simulink model "sender"  (R2019b)
settings: Solver=VariableStepAuto  StartTime=0.0  StopTime=10e-3  RelTol=1e-3
values from neighbouring files (symbols this model uses):
  f_c = 100e3    (= 100000)    [loopFil.m]
  filter = rcosdesign(alpha,symNum,sym,'sqrt')    [loopFil.m]    (also in rcosfilter.m)
  Gc = 1    [loopFil.m]
  Gg = 1.5    [loopFil.m]
  inc = 2^16*f_nco/Fs    (= 5688.88888889)    [loopFil.m]
  inc2 = 2^16*f_nco2/Fs    (= 8533.33333333)    [loopFil.m]
  inc_src = 2^16*f_src/Fs    (= 1092.26666667)    [loopFil.m]
undefined symbols (not defined in the file or in its folder): ac, ag, bc, bg, fdesignblkfcn, gcbh
libraries: dspsigops x22, dspsrcs4 x8, simulink x4
settings Model: Creator=Administrator  LastModifiedBy=Administrator

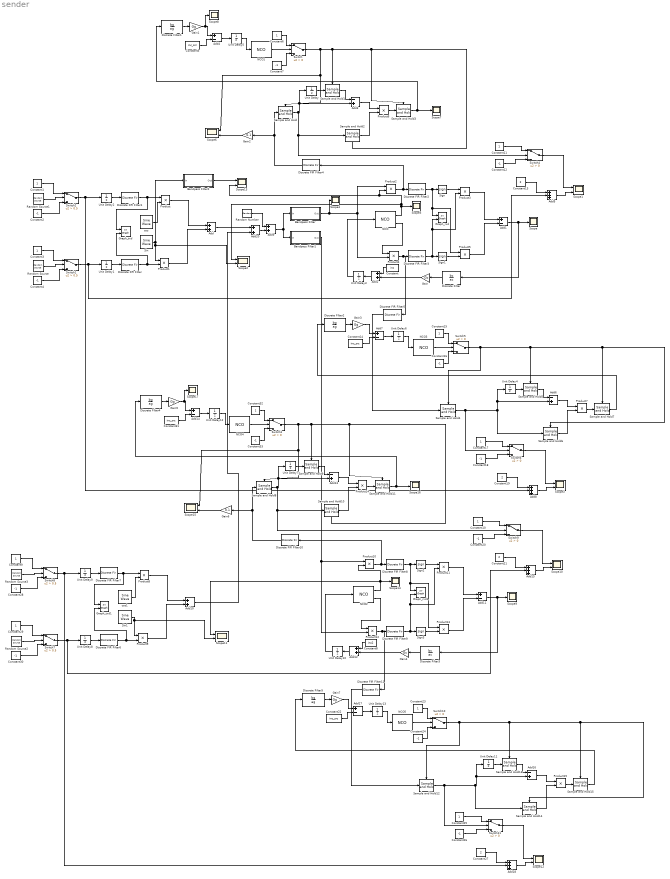
== system sender ==
  Add{,2,10,12} (4 alike) : Sum
  Add1 : Sum  Inputs=+-
  Add11 : Sum  Inputs=+-
  Add{3,6,13,16} (4 alike) : Sum  Inputs=-+
  Add{4,7,14,17} (4 alike) : Sum  Inputs=+-  OutDataTypeStr=int16
  Add{5,8,15,18} (4 alike) : Sum  Inputs=+++  OutDataTypeStr=int16
  Add20 : Sum  OutDataTypeStr=int16
  Add9 : Sum  OutDataTypeStr=int16
  Bandpass Filter : Subsystem  DialogController=fdesignblkfcn  InitFcn=fdesignblkfcn(gcbh, {'InitFcn'});  mask(Bandpass Filter){}
      mask help: Design a bandpass filter
      settings: CopyFcn=fdesignblkfcn(gcbh, {'CopyFcn'});
      mask Help: helpview(mapfilelocation('dsp'), 'dspbandpassfilter');
      mask Display: disp('Bandpass');
  Bandpass Filter1 : Subsystem  DialogController=fdesignblkfcn  InitFcn=fdesignblkfcn(gcbh, {'InitFcn'});  mask(Bandpass Filter){}
      mask help: Design a bandpass filter
      settings: CopyFcn=fdesignblkfcn(gcbh, {'CopyFcn'});
      mask Help: helpview(mapfilelocation('dsp'), 'dspbandpassfilter');
      mask Display: disp('Bandpass');
  Bandpass Filter2 : Subsystem  DialogController=fdesignblkfcn  InitFcn=fdesignblkfcn(gcbh, {'InitFcn'});  mask(Bandpass Filter){}
      mask help: Design a bandpass filter
      settings: CopyFcn=fdesignblkfcn(gcbh, {'CopyFcn'});
      mask Help: helpview(mapfilelocation('dsp'), 'dspbandpassfilter');
      mask Display: disp('Bandpass');
  Constant : Constant  Value=inc  OutDataTypeStr=int16  SampleTime=1/(60*19.2e3)
  Constant{1,3,6,9..11,15,17,23,25,29,32} (12 alike) : Constant  SampleTime=1/(60*19.2e3)
  Constant{2,4,7,12,16,18,20,24,26,28,30,33} (12 alike) : Constant  Value=-1  SampleTime=1/(60*19.2e3)
  Constant{13,19,21,27} (4 alike) : Constant  Value=2  SampleTime=1/(60*19.2e3)
  Constant{5,14,22,31} (4 alike) : Constant  Value=inc_src  OutDataTypeStr=int32  SampleTime=1/(60*19.2e3)
  Constant8 : Constant  Value=inc2  OutDataTypeStr=int16  SampleTime=1/(60*19.2e3)
  Discrete FIR Filter{,1..11} (12 alike) : DiscreteFir  Coefficients=filter
  Discrete Filter : DiscreteFilter  Numerator=bc  Denominator=ac
  Discrete Filter{1..2,4..5} (4 alike) : DiscreteFilter  Numerator=bg  Denominator=ag
  Discrete Filter3 : DiscreteFilter  Numerator=bc  Denominator=ac
  Gain : Gain  Gain=Gc  OutDataTypeStr=int16
  Gain{1,3,5,7} (4 alike) : Gain  Gain=Gg
  Gain2 : Gain  Gain=0.1
  Gain4 : Gain  Gain=Gc  OutDataTypeStr=int16
  Gain6 : Gain  Gain=0.1
  Graph_rxd : simulink/Sinks/XY Graph  xmin=-50  xmax=50  ymin=-50  ymax=50  st=-1
  Graph_rxd1 : simulink/Sinks/XY Graph  xmin=-50  xmax=50  ymin=-50  ymax=50  st=-1
  Graph_txd : simulink/Sinks/XY Graph  xmin=-16  xmax=16  ymin=-16  ymax=16  st=-1
  Graph_txd1 : simulink/Sinks/XY Graph  xmin=-16  xmax=16  ymin=-16  ymax=16  st=-1
  NCO : dspsigops/NCO  AccIncSrc=Input port  AccInc=100  PhaseOffsetSrc=Specify via dialog  PhaseOffset=0  AccumWL=16  HasDither=on  DitherWL=4  PNgeneratorLength=19  HasPhaseQuantizer=on  TableDepth=12  HasOutputPhaseError=off  Formula=Sine and cosine  DataType=single  OutputWL=16  OutputFL=14  CompMethod=Table lookup (no interpolation)  SampleTime=1  SamplesPerFrame=1  OutputFrames=off
      settings: SourceProductName=DSP System Toolbox  SourceProductBaseCode=DS
  NCO{1,3..5} (4 alike) : dspsigops/NCO  AccIncSrc=Input port  AccInc=100  PhaseOffsetSrc=Specify via dialog  PhaseOffset=0  AccumWL=16  HasDither=on  DitherWL=4  PNgeneratorLength=19  HasPhaseQuantizer=on  TableDepth=12  HasOutputPhaseError=off  Formula=Sine  DataType=single  OutputWL=16  OutputFL=14  CompMethod=Table lookup (no interpolation)  SampleTime=1  SamplesPerFrame=1  OutputFrames=off
      settings: SourceProductName=DSP System Toolbox  SourceProductBaseCode=DS
  NCO2 : dspsigops/NCO  AccIncSrc=Input port  AccInc=100  PhaseOffsetSrc=Specify via dialog  PhaseOffset=0  AccumWL=16  HasDither=on  DitherWL=4  PNgeneratorLength=19  HasPhaseQuantizer=on  TableDepth=12  HasOutputPhaseError=off  Formula=Sine and cosine  DataType=single  OutputWL=16  OutputFL=14  CompMethod=Table lookup (no interpolation)  SampleTime=1  SamplesPerFrame=1  OutputFrames=off
      settings: SourceProductName=DSP System Toolbox  SourceProductBaseCode=DS
  Product{,1..15} (16 alike) : Product
  Random Number : RandomNumber  Variance=0  SampleTime=1/(60*19.2e3)
  Random Source{,1..3} (4 alike) : dspsrcs4/Random Source  SrcType=Uniform  NormMethod=Ziggurat  CltLength=12  MinVal=0  MaxVal=1  MeanVal=0  VarVal=1  RepMode=Not repeatable  rawSeed=1  IsInherit=off  SampMode=Discrete  SampTime=1/(19.2e3)  SampFrame=1  DataType=Double  OutComplex=Real  OutputFrames=off
  Sample and Hold{,1,4..5,8..9,12..13} (8 alike) : dspsigops/Sample and Hold  trig=Rising edge  initCond=0  latchinput=off
  Sample and Hold{2,6,10,14} (4 alike) : dspsigops/Sample and Hold  trig=Falling edge  initCond=0  latchinput=off
  Sample and Hold{3,7,11,15} (4 alike) : dspsigops/Sample and Hold  Tag=error  trig=Rising edge  initCond=0  latchinput=off
  Scope{,4..5,7..9,14,16..17} (9 alike) : Scope
  Scope{1..3,6,10..13,15} (9 alike) : Scope  NumInputPorts=2
  Sign{,1..3} (4 alike) : Signum
  Sin : dspsrcs4/Sine Wave  Amplitude=1  Frequency=f_c  Phase=0  SampleMode=Discrete  OutComplex=Real  CompMethod=Trigonometric fcn  TableSize=Speed  SampleTime=1/(60*19.2e3)  SamplesPerFrame=1  ResetState=Restart at time zero  OutputFrames=off  dataType=double  wordLen=16  udDataType=sfix(16)  fracBitsMode=Best precision  numFracBits=15  OutDataTypeStr=double  LastOutDataTypeStr=double
  Sin1 : dspsrcs4/Sine Wave  Amplitude=1  Frequency=150e3  Phase=0  SampleMode=Discrete  OutComplex=Real  CompMethod=Trigonometric fcn  TableSize=Speed  SampleTime=1/(60*19.2e3)  SamplesPerFrame=1  ResetState=Restart at time zero  OutputFrames=off  dataType=double  wordLen=16  udDataType=sfix(16)  fracBitsMode=Best precision  numFracBits=15  OutDataTypeStr=double  LastOutDataTypeStr=double
  Switch{,3..6,9..11} (8 alike) : Switch  Criteria=u2 > Threshold
  Switch{1..2,7..8} (4 alike) : Switch  Criteria=u2 > Threshold  Threshold=0.5
  Unit Delay{,1..13} (14 alike) : UnitDelay  SampleTime=-1  HasFrameUpgradeWarning=on
  cos : dspsrcs4/Sine Wave  Amplitude=1  Frequency=f_c  Phase=pi/2  SampleMode=Discrete  OutComplex=Real  CompMethod=Trigonometric fcn  TableSize=Speed  SampleTime=1/(60*19.2e3)  SamplesPerFrame=1  ResetState=Restart at time zero  OutputFrames=off  dataType=double  wordLen=16  udDataType=sfix(16)  fracBitsMode=Best precision  numFracBits=15  OutDataTypeStr=double  LastOutDataTypeStr=double
  cos1 : dspsrcs4/Sine Wave  Amplitude=1  Frequency=150e3  Phase=pi/2  SampleMode=Discrete  OutComplex=Real  CompMethod=Trigonometric fcn  TableSize=Speed  SampleTime=1/(60*19.2e3)  SamplesPerFrame=1  ResetState=Restart at time zero  OutputFrames=off  dataType=double  wordLen=16  udDataType=sfix(16)  fracBitsMode=Best precision  numFracBits=15  OutDataTypeStr=double  LastOutDataTypeStr=double
  wires:
  Unit Delay1/1 -> Discrete FIR Filter/1
  Discrete FIR Filter/1 -> Graph_txd/2, Product1/2
  Sin/1 -> Bandpass Filter2/1(In), Scope2/2, Product1/1
  cos/1 -> Product/2
  Product/1 -> Add/1
  Product1/1 -> Add/2
  Product3/1 -> Add1/1
  Sign1/1 -> Product5/2
  Product5/1 -> Add1/2
  Discrete FIR Filter2/1 -> Graph_rxd/1, Product5/1, Sign/1
  Discrete FIR Filter3/1 -> Graph_rxd/2, Product3/2, Sign1/1
  Sign/1 -> Product3/1
  Add1/1 -> Discrete Filter/1, Scope/1
  Product2/1 -> Discrete FIR Filter4/1, Discrete FIR Filter2/1
  Product4/1 -> Discrete FIR Filter5/1, Discrete FIR Filter3/1
  NCO/1 -> Scope13/2, Product2/2, Scope2/1, Scope5/1
  NCO/2 -> Product4/1
  Constant/1 -> Add2/1
  Add2/1 -> Unit Delay3/1
  Unit Delay3/1 -> NCO/1
  Sample and Hold/1 -> Sample and Hold2/1, Switch4/2, Unit Delay/1, Add3/2
  Gain1/1 -> Scope8/1, Add4/1
  Switch/1 -> Sample and Hold1/Trigger, Sample and Hold2/Trigger, Sample and Hold3/Trigger, Sample and Hold/Trigger, Scope6/1
  Constant6/1 -> Switch/1
  Sample and Hold1/1 -> Add3/1
  Product6/1 -> Sample and Hold3/1
  Unit Delay5/1 -> NCO1/1
  NCO1/1 -> Switch/2
  Constant5/1 -> Add4/2
  Constant7/1 -> Switch/3
  Unit Delay/1 -> Sample and Hold1/1
  Sample and Hold2/1 -> Product6/2
  Add4/1 -> Unit Delay5/1
  Add3/1 -> Product6/1
  Discrete Filter/1 -> Gain/1
  Gain/1 -> Add2/2
  Discrete Filter1/1 -> Gain1/1
  Sample and Hold3/1 -> Scope7/1, Discrete Filter1/1
  Discrete FIR Filter4/1 -> Sample and Hold/1, Gain2/1
  Constant1/1 -> Switch2/1
  Constant2/1 -> Switch2/3
  Random Source1/1 -> Switch2/2
  Constant3/1 -> Switch1/1
  Constant4/1 -> Switch1/3
  Random Source/1 -> Switch1/2
  Gain2/1 -> Scope6/2
  Switch2/1 -> Add8/2, Unit Delay2/1
  Switch1/1 -> Add5/2, Unit Delay1/1
  Constant11/1 -> Switch4/1
  Constant12/1 -> Switch4/3
  Switch4/1 -> Scope1/1
  Constant13/1 -> Add5/1
  Add5/1 -> Scope1/2
  Constant14/1 -> Add7/2
  Sample and Hold7/1 -> Discrete Filter2/1
  Discrete Filter2/1 -> Gain3/1
  Add7/1 -> Unit Delay6/1
  Discrete FIR Filter5/1 -> Sample and Hold4/1
  Unit Delay4/1 -> Sample and Hold5/1
  Sample and Hold6/1 -> Product7/2
  Product7/1 -> Sample and Hold7/1
  Add6/1 -> Product7/1
  Gain3/1 -> Add7/1
  Constant16/1 -> Switch5/3
  Unit Delay6/1 -> NCO3/1
  Switch5/1 -> Sample and Hold5/Trigger, Sample and Hold6/Trigger, Sample and Hold7/Trigger, Sample and Hold4/Trigger
  NCO3/1 -> Switch5/2
  Sample and Hold4/1 -> Switch6/2, Sample and Hold6/1, Unit Delay4/1, Add6/2
  Sample and Hold5/1 -> Add6/1
  Constant15/1 -> Switch5/1
  Constant18/1 -> Switch6/3
  Switch6/1 -> Scope3/1
  Constant17/1 -> Switch6/1
  Add8/1 -> Scope3/2
  Constant19/1 -> Add8/1
  Random Number/1 -> Add9/1
  Constant24/1 -> Switch10/3
  Constant23/1 -> Switch10/1
  Switch9/1 -> Scope10/1
  Constant10/1 -> Switch9/1
  Product15/1 -> Sample and Hold15/1
  Add16/1 -> Product15/1
  Sample and Hold14/1 -> Product15/2
  Discrete FIR Filter11/1 -> Sample and Hold12/1
  Add17/1 -> Unit Delay13/1
  Sample and Hold15/1 -> Discrete Filter5/1
  Constant21/1 -> Add15/1
  NCO5/1 -> Switch10/2
  Unit Delay13/1 -> NCO5/1
  Sample and Hold10/1 -> Product14/2
  Constant31/1 -> Add14/2
  Discrete Filter3/1 -> Gain4/1
  Gain5/1 -> Scope17/1, Add14/1
  Constant9/1 -> Switch8/1
  Constant29/1 -> Switch7/1
  Discrete Filter4/1 -> Gain5/1
  Constant28/1 -> Switch8/3
  Constant30/1 -> Switch7/3
  Sign2/1 -> Product11/1
  Product10/1 -> Discrete FIR Filter10/1, Discrete FIR Filter8/1
  Discrete FIR Filter7/1 -> Graph_txd1/1, Product8/1
  Random Source2/1 -> Switch7/2
  Unit Delay8/1 -> Discrete FIR Filter6/1
  Random Source3/1 -> Switch8/2
  Add14/1 -> Unit Delay12/1
  Switch8/1 -> Add18/2, Unit Delay9/1
  Discrete FIR Filter10/1 -> Sample and Hold8/1, Gain6/1
  Unit Delay7/1 -> Sample and Hold9/1
  Constant8/1 -> Add12/1
  Constant32/1 -> Switch3/1
  Product11/1 -> Add11/1
  Product14/1 -> Sample and Hold11/1
  Gain4/1 -> Add12/2
  Add13/1 -> Product14/1
  Constant22/1 -> Add17/2
  Discrete FIR Filter9/1 -> Graph_rxd1/2, Product11/2, Sign3/1
  Add12/1 -> Unit Delay10/1
  Unit Delay12/1 -> NCO4/1
  Discrete FIR Filter8/1 -> Graph_rxd1/1, Product13/1, Sign2/1
  Product12/1 -> Discrete FIR Filter11/1, Discrete FIR Filter9/1
  NCO4/1 -> Switch3/2
  Switch3/1 -> Sample and Hold9/Trigger, Sample and Hold10/Trigger, Sample and Hold11/Trigger, Sample and Hold8/Trigger, Scope15/1
  NCO2/1 -> Scope11/1, Scope14/1, Product10/2
  Product9/1 -> Add10/2
  Gain6/1 -> Scope15/2
  Unit Delay10/1 -> NCO2/1
  Add11/1 -> Discrete Filter3/1, Scope9/1
  Discrete FIR Filter6/1 -> Graph_txd1/2, Product9/2
  Product8/1 -> Add10/1
  Constant20/1 -> Switch9/3
  Sample and Hold8/1 -> Sample and Hold10/1, Switch9/2, Unit Delay7/1, Add13/2
  Sample and Hold11/1 -> Scope16/1, Discrete Filter4/1
  Sample and Hold13/1 -> Add16/1
  Gain7/1 -> Add17/1
  Unit Delay9/1 -> Discrete FIR Filter7/1
  NCO2/2 -> Product12/1
  Sample and Hold12/1 -> Switch11/2, Sample and Hold14/1, Unit Delay11/1, Add16/2
  Switch10/1 -> Sample and Hold13/Trigger, Sample and Hold14/Trigger, Sample and Hold15/Trigger, Sample and Hold12/Trigger
  Sign3/1 -> Product13/2
  Sample and Hold9/1 -> Add13/1
  Constant33/1 -> Switch3/3
  Unit Delay11/1 -> Sample and Hold13/1
  Constant26/1 -> Switch11/3
  Constant27/1 -> Add18/1
  Add10/1 -> Add20/2
  cos1/1 -> Product8/2
  Add15/1 -> Scope10/2
  Discrete Filter5/1 -> Gain7/1
  Switch7/1 -> Add15/2, Unit Delay8/1
  Switch11/1 -> Scope12/1
  Add18/1 -> Scope12/2
  Product13/1 -> Add11/2
  Sin1/1 -> Scope11/2, Product9/1
  Constant25/1 -> Switch11/1
  Add/1 -> Add20/1
  Add20/1 -> Add9/2
  Add9/1 -> Bandpass Filter1/1(In), Bandpass Filter/1(In)
  Bandpass Filter/1(Out) -> Scope4/1, Product4/2, Product2/1
  Bandpass Filter1/1(Out) -> Product12/2, Product10/1
  Unit Delay2/1 -> Discrete FIR Filter1/1
  Discrete FIR Filter1/1 -> Graph_txd/1, Product/1
  Bandpass Filter2/1(Out) -> Scope13/1

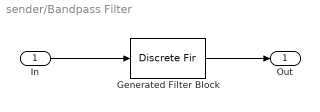
== system sender/Bandpass Filter ==
  In : Inport
  Generated Filter Block : DiscreteFir  Tag=BlockMethodSubSystem  Coefficients=[-0.00447663543698568339 0.000909734626442467928 0.00103144091472800493 0.00117150934759783273 0.00122541528560887909 0.00113510661548536004 0.000909996327315583213 0.000626249819161312296 0.000386976186586897655 0.000275236287237889607 0.000305293995293338082 0.000410885729691512665 0.000465656888105368816 0.000344741554262389428 -8.84306575163300301e-06 -0.000532306766293209194 -0.00104196374405414027 -0.0012942895075897104 -0.00105718581011491133 -0.00028545139796183356 0.000901840536366371563 0.00216487357221187022 0.00304036871182613569 0.00311027057233250999 0.00216017320961272175 0.000307885195072063467 -0.0019879902221413958 -0.00402860133366981198 -0.0050944160846013338 -0.00468824297124444556 -0.00274596641431512026 0.000294848123827263012 0.00357917401808327887 0.00608773505009416009 0.00695426055454248689 0.00578049004676658117 0.00278379966576174434 -0.00120555896175186632 -0.00500621249491005598 -0.00744335977347669424 -0.00773446500257566304 -0.0057554264274766679 -0.00209888582102140146 0.00211378112926276056 0.00559370238698311557 0.00731153298323194197 0.0068289943222984489 0.0044322068824486742 0.00100641956520797216 -0.00228949122629135355 -0.00444187653465884756 -0.00492936632583139585 -0.00387813164332000181 -0.00196665383254771876 -0.000112645078908951181 0.000918610299865273497 0.000840290520142906658 -3.28752332547652473e-05 -0.000937381809383888188 -0.00101593506765935027 0.000247188816189225329 0.00270940840555784681 0.00550769313755324411 0.00732407434924705909 0.00689282494380578231 0.0035837751881583539 -0.00218509637750114588 -0.00888523185488331035 -0.0142586802133901173 -0.0160439725077658295 -0.0128357463896090034 -0.00474928297943181567 0.00635955123611510638 0.0172848205266944305 0.0243889437313596288 0.0247969669475410943 0.0174728508642247385 0.00379519144498540557 -0.0126279108671645407 -0.0269086705440964094 -0.0343525427302637243 -0.0319993184595248545 -0.0197306013734877342 -0.000537171077681756343 0.0201983892437221924 0.0362412828216668315 0.0424144111232741955 0.0362849010571170347 0.0190728390775604766 -0.00455029963286844238 -0.0277569751717750557 -0.0435860166716085101 -0.04708132819489734 -0.0368717023030117955 -0.0156820368904130036 0.0104096904379330536 0.0337639655314302123 0.0474773110556236874 0.0474773110556236874 0.0337639655314302123 0.0104096904379330536 -0.0156820368904130036 -0.0368717023030117955 -0.04708132819489734 -0.0435860166716085101 -0.0277569751717750557 -0.00455029963286844238 0.0190728390775604766 0.0362849010571170347 0.0424144111232741955 0.0362412828216668315 0.0201983892437221924 -0.000537171077681756343 -0.0197306013734877342 -0.0319993184595248545 -0.0343525427302637243 -0.0269086705440964094 -0.0126279108671645407 0.00379519144498540557 0.0174728508642247385 0.0247969669475410943 0.0243889437313596288 0.0172848205266944305 0.00635955123611510638 -0.00474928297943181567 -0.0128357463896090034 -0.0160439725077658295 -0.0142586802133901173 -0.00888523185488331035 -0.00218509637750114588 0.0035837751881583539 0.00689282494380578231 0.00732407434924705909 0.00550769313755324411 0.00270940840555784681 0.000247188816189225329 -0.00101593506765935027 -0.000937381809383888188 -3.28752332547652473e-05 0.000840290520142906658 0.000918610299865273497 -0.000112645078908951181 -0.00196665383254771876 -0.00387813164332000181 -0.00492936632583139585 -0.00444187653465884756 -0.00228949122629135355 0.00100641956520797216 0.0044322068824486742 0.0068289943222984489 0.00731153298323194197 0.00559370238698311557 0.00211378112926276056 -0.00209888582102140146 -0.0057554264274766679 -0.00773446500257566304 -0.00744335977347669424 -0.00500621249491005598 -0.00120555896175186632 0.00278379966576174434 0.00578049004676658117 0.00695426055454248689 0.00608773505009416009 0.00357917401808327887 0.000294848123827263012 -0.00274596641431512026 -0.00468824297124444556 -0.0050944160846013338 -0.00402860133366981198 -0.0019879902221413958 0.000307885195072063467 ...(+593 chars)]  InputProcessing=Columns as channels (frame based)
  Out : Outport  VectorParamsAs1DForOutWhenUnconnected=off
  wires:
  In/1 -> Generated Filter Block/1
  Generated Filter Block/1 -> Out/1

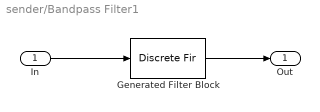
== system sender/Bandpass Filter1 ==
  In : Inport
  Generated Filter Block : DiscreteFir  Tag=BlockMethodSubSystem  Coefficients=[-0.00513283775238465838 -0.000260973964489737489 0.000148020415231001935 0.000510520486361654494 0.000585311315873687267 0.000357927338053887906 4.78096091557521016e-05 -0.000101141168061158644 -2.40549056035486639e-05 0.000104438492814411775 6.33944054583210348e-05 -0.000184314439572696477 -0.000383082099035147138 -0.000197897778972161778 0.000470661980938358142 0.00122838918138592091 0.00141323508092730879 0.000617811338810364541 -0.000907813208907811559 -0.00218946120403817543 -0.00216111712363519642 -0.000467631398896839641 0.00205690913425946812 0.00376061955269577086 0.0032332776314513605 0.000411762971910405 -0.00312697743076167066 -0.0050269882673527836 -0.00372585899418415587 0.000320592717748089881 0.004700701266069085 0.00647983507549126925 0.00419492006089576368 -0.000994697068408854652 -0.00587294605981605877 -0.00718885955841396147 -0.00386829146078710405 0.00214025510169020463 0.00702216197553551594 0.00758398704586064985 0.00339460320059374338 -0.00287456802689214398 -0.00720081882678116816 -0.00687074018474427735 -0.00225752365525445659 0.00351336575122772245 0.00673946669246123717 0.00561333018014949572 0.00129780683282472963 -0.00310330157040250056 -0.00482844820072750661 -0.00330353492577721477 -0.000248405096492162504 0.0019089041498641145 0.00197691282864936695 0.000760454530839100792 7.09912362974809974e-05 0.000889860457378048759 0.00229964635916493155 0.0022174724366619031 -0.000580178143692883751 -0.00483185255428195473 -0.00717623205211899515 -0.00462195267532225854 0.00263274057460825004 0.0103849104759527223 0.0127698646208553035 0.006522027818665262 -0.00585659328937262851 -0.0167321121933305429 -0.0180017918165207846 -0.00696813786083315054 0.0107580790731426137 0.0239322396744394358 0.0228047317577795873 0.00618991382168822268 -0.0165889741586470567 -0.0308660825058385546 -0.0261128295753231335 -0.00357196739022629453 0.0234268963018055276 0.037371854357786366 0.027998113293169348 -0.000265427844694192134 -0.0301811585580043923 -0.0423030515170038507 -0.0277166471058265078 0.00548812527473336795 0.0366765859508899131 0.045623766484546302 0.0257532339130446507 -0.011085525408748716 -0.0417482129883886971 -0.0464974348902534168 -0.021843570468083974 0.0169210297206139615 0.0453172034078331218 0.0453172034078331218 0.0169210297206139615 -0.021843570468083974 -0.0464974348902534168 -0.0417482129883886971 -0.011085525408748716 0.0257532339130446507 0.045623766484546302 0.0366765859508899131 0.00548812527473336795 -0.0277166471058265078 -0.0423030515170038507 -0.0301811585580043923 -0.000265427844694192134 0.027998113293169348 0.037371854357786366 0.0234268963018055276 -0.00357196739022629453 -0.0261128295753231335 -0.0308660825058385546 -0.0165889741586470567 0.00618991382168822268 0.0228047317577795873 0.0239322396744394358 0.0107580790731426137 -0.00696813786083315054 -0.0180017918165207846 -0.0167321121933305429 -0.00585659328937262851 0.006522027818665262 0.0127698646208553035 0.0103849104759527223 0.00263274057460825004 -0.00462195267532225854 -0.00717623205211899515 -0.00483185255428195473 -0.000580178143692883751 0.0022174724366619031 0.00229964635916493155 0.000889860457378048759 7.09912362974809974e-05 0.000760454530839100792 0.00197691282864936695 0.0019089041498641145 -0.000248405096492162504 -0.00330353492577721477 -0.00482844820072750661 -0.00310330157040250056 0.00129780683282472963 0.00561333018014949572 0.00673946669246123717 0.00351336575122772245 -0.00225752365525445659 -0.00687074018474427735 -0.00720081882678116816 -0.00287456802689214398 0.00339460320059374338 0.00758398704586064985 0.00702216197553551594 0.00214025510169020463 -0.00386829146078710405 -0.00718885955841396147 -0.00587294605981605877 -0.000994697068408854652 0.00419492006089576368 0.00647983507549126925 0.004700701266069085 0.000320592717748089881 -0.00372585899418415587 -0.0050269882673527836 -0.00312697743076167066 0.000411762971910405 0.0032332776314513605 0.00376061955269577086 0.00205690913425946812 ...(+534 chars)]  InputProcessing=Columns as channels (frame based)
  Out : Outport  VectorParamsAs1DForOutWhenUnconnected=off
  wires:
  In/1 -> Generated Filter Block/1
  Generated Filter Block/1 -> Out/1

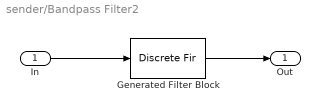
== system sender/Bandpass Filter2 ==
  In : Inport
  Generated Filter Block : DiscreteFir  Tag=BlockMethodSubSystem  Coefficients=[-0.00447663543698568339 0.000909734626442467928 0.00103144091472800493 0.00117150934759783273 0.00122541528560887909 0.00113510661548536004 0.000909996327315583213 0.000626249819161312296 0.000386976186586897655 0.000275236287237889607 0.000305293995293338082 0.000410885729691512665 0.000465656888105368816 0.000344741554262389428 -8.84306575163300301e-06 -0.000532306766293209194 -0.00104196374405414027 -0.0012942895075897104 -0.00105718581011491133 -0.00028545139796183356 0.000901840536366371563 0.00216487357221187022 0.00304036871182613569 0.00311027057233250999 0.00216017320961272175 0.000307885195072063467 -0.0019879902221413958 -0.00402860133366981198 -0.0050944160846013338 -0.00468824297124444556 -0.00274596641431512026 0.000294848123827263012 0.00357917401808327887 0.00608773505009416009 0.00695426055454248689 0.00578049004676658117 0.00278379966576174434 -0.00120555896175186632 -0.00500621249491005598 -0.00744335977347669424 -0.00773446500257566304 -0.0057554264274766679 -0.00209888582102140146 0.00211378112926276056 0.00559370238698311557 0.00731153298323194197 0.0068289943222984489 0.0044322068824486742 0.00100641956520797216 -0.00228949122629135355 -0.00444187653465884756 -0.00492936632583139585 -0.00387813164332000181 -0.00196665383254771876 -0.000112645078908951181 0.000918610299865273497 0.000840290520142906658 -3.28752332547652473e-05 -0.000937381809383888188 -0.00101593506765935027 0.000247188816189225329 0.00270940840555784681 0.00550769313755324411 0.00732407434924705909 0.00689282494380578231 0.0035837751881583539 -0.00218509637750114588 -0.00888523185488331035 -0.0142586802133901173 -0.0160439725077658295 -0.0128357463896090034 -0.00474928297943181567 0.00635955123611510638 0.0172848205266944305 0.0243889437313596288 0.0247969669475410943 0.0174728508642247385 0.00379519144498540557 -0.0126279108671645407 -0.0269086705440964094 -0.0343525427302637243 -0.0319993184595248545 -0.0197306013734877342 -0.000537171077681756343 0.0201983892437221924 0.0362412828216668315 0.0424144111232741955 0.0362849010571170347 0.0190728390775604766 -0.00455029963286844238 -0.0277569751717750557 -0.0435860166716085101 -0.04708132819489734 -0.0368717023030117955 -0.0156820368904130036 0.0104096904379330536 0.0337639655314302123 0.0474773110556236874 0.0474773110556236874 0.0337639655314302123 0.0104096904379330536 -0.0156820368904130036 -0.0368717023030117955 -0.04708132819489734 -0.0435860166716085101 -0.0277569751717750557 -0.00455029963286844238 0.0190728390775604766 0.0362849010571170347 0.0424144111232741955 0.0362412828216668315 0.0201983892437221924 -0.000537171077681756343 -0.0197306013734877342 -0.0319993184595248545 -0.0343525427302637243 -0.0269086705440964094 -0.0126279108671645407 0.00379519144498540557 0.0174728508642247385 0.0247969669475410943 0.0243889437313596288 0.0172848205266944305 0.00635955123611510638 -0.00474928297943181567 -0.0128357463896090034 -0.0160439725077658295 -0.0142586802133901173 -0.00888523185488331035 -0.00218509637750114588 0.0035837751881583539 0.00689282494380578231 0.00732407434924705909 0.00550769313755324411 0.00270940840555784681 0.000247188816189225329 -0.00101593506765935027 -0.000937381809383888188 -3.28752332547652473e-05 0.000840290520142906658 0.000918610299865273497 -0.000112645078908951181 -0.00196665383254771876 -0.00387813164332000181 -0.00492936632583139585 -0.00444187653465884756 -0.00228949122629135355 0.00100641956520797216 0.0044322068824486742 0.0068289943222984489 0.00731153298323194197 0.00559370238698311557 0.00211378112926276056 -0.00209888582102140146 -0.0057554264274766679 -0.00773446500257566304 -0.00744335977347669424 -0.00500621249491005598 -0.00120555896175186632 0.00278379966576174434 0.00578049004676658117 0.00695426055454248689 0.00608773505009416009 0.00357917401808327887 0.000294848123827263012 -0.00274596641431512026 -0.00468824297124444556 -0.0050944160846013338 -0.00402860133366981198 -0.0019879902221413958 0.000307885195072063467 ...(+593 chars)]  InputProcessing=Columns as channels (frame based)
  Out : Outport  VectorParamsAs1DForOutWhenUnconnected=off
  wires:
  In/1 -> Generated Filter Block/1
  Generated Filter Block/1 -> Out/1
